simulink model "ClosedLoop_Test"  (R2022b)
settings: Solver=VariableStepAuto  StartTime=0.0  StopTime=10.0  RelTol=1e-3
libraries: cstblocks x7
settings Model: Creator=antoninrenoir  LastModifiedBy=emili

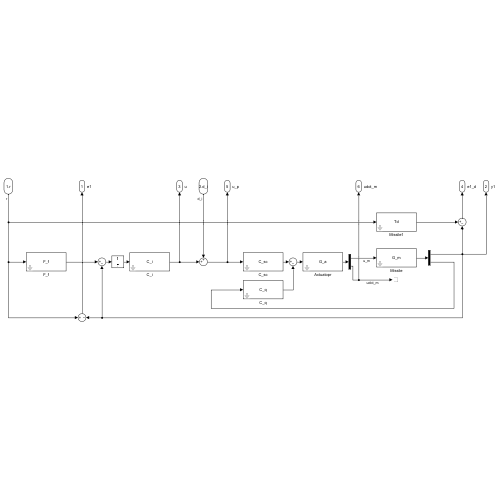
[thumbnail: Simulink's stored preview of the top-level diagram]
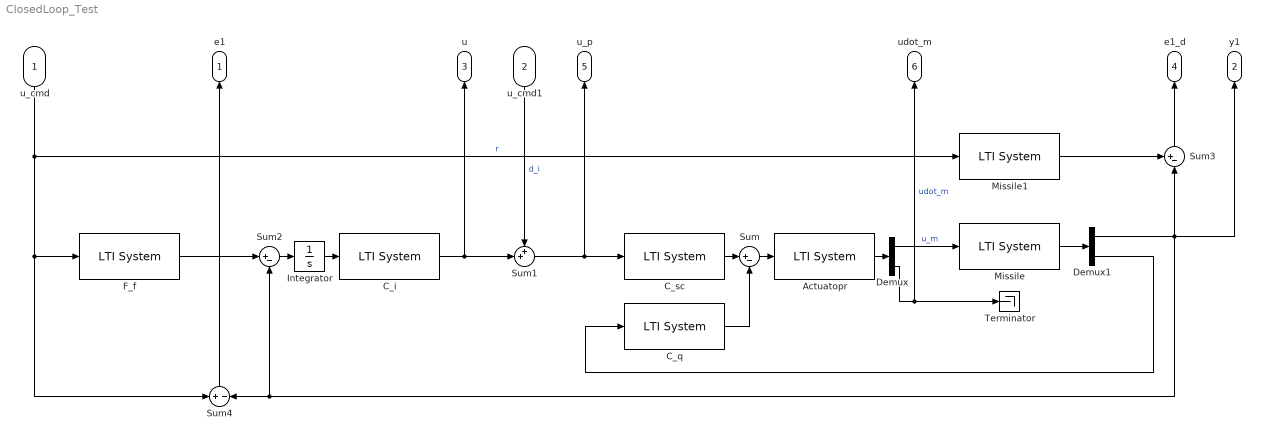
== system ClosedLoop_Test ==
  u_cmd : Inport
  u_cmd1 : Inport  Port=2
  Actuatopr : cstblocks/LTI System  sys=G_a  IC=[]
  C_i : cstblocks/LTI System  sys=C_i  IC=[]
  C_q : cstblocks/LTI System  sys=C_q  IC=[]
  C_sc : cstblocks/LTI System  sys=C_sc  IC=[]
  Demux : Demux  Outputs=2
  Demux1 : Demux  Outputs=2
  F_f : cstblocks/LTI System  sys=F_f  IC=[]
  Integrator : Integrator
  Missile : cstblocks/LTI System  sys=G_m  IC=[]
  Missile1 : cstblocks/LTI System  sys=Td  IC=[]
  Sum : Sum  Inputs=|+-
  Sum1 : Sum  Inputs=++|
  Sum2 : Sum  Inputs=|+-
  Sum3 : Sum  Inputs=+-|
  Sum4 : Sum  Inputs=+|-
  Terminator : Terminator
  e1 : Outport
  y1 : Outport  Port=2
  u : Outport  Port=3
  e1_d : Outport  Port=4
  u_p : Outport  Port=5
  udot_m : Outport  Port=6
  wires:
  Actuatopr/1 -> Demux/1
  C_q/1 -> Sum/2
  Demux/2 -> udot_m/1, Terminator/1  "udot_m"
  Demux/1 -> Missile/1  "u_m"
  Sum/1 -> Actuatopr/1
  Missile/1 -> Demux1/1
  Integrator/1 -> C_i/1
  C_sc/1 -> Sum/1
  Demux1/2 -> C_q/1
  Sum1/1 -> u_p/1, C_sc/1
  C_i/1 -> Sum1/2, u/1
  Sum2/1 -> Integrator/1
  u_cmd/1 -> Sum4/1, F_f/1, Missile1/1  "r"
  Demux1/1 -> y1/1, Sum4/2, Sum2/2, Sum3/2
  Missile1/1 -> Sum3/1
  Sum3/1 -> e1_d/1
  F_f/1 -> Sum2/1
  Sum4/1 -> e1/1
  u_cmd1/1 -> Sum1/1  "d_i"
